simulink model "Vector_xFFT_Ex2"  (R2025a)
settings: Solver=ode45  StartTime=0.0  StopTime=4096/20e3  RelTol=1e-3  EnableMultiTasking=on
undefined symbols (not defined in the file): i, L, vsva1596, xcvc1502
libraries: hdlBasic x7, hdlSSR x5, dspsrcs4 x3, dspxfrm3 x1, vmcUtilities x1
settings Model: Creator=dahlawat  LastModifiedBy=sdegala
settings SolverCC: AlgebraicLoopSolver=TrustRegion
settings DataIOCC: LimitDataPoints=on  SaveFormat=Array  ReturnWorkspaceOutputs=off
settings OptimizationCC: LifeSpan=inf
settings DebuggingCC: UnderspecifiedInitializationDetection=Classic  MergeDetectMultiDrivingBlocksExec=none  SolverPrmCheckMsg=warning  UnconnectedInputMsg=warning  UnconnectedOutputMsg=warning  UnconnectedLineMsg=warning  StateNameClashWarn=warning  SFUnexpectedBacktrackingDiag=warning  SFNoUnconditionalDefaultTransitionDiag=warning  SFExecutionAtInitializationDiag=none  ArithmeticOperatorsInVariantConditions=warning
settings HardwareCC: ProdBitPerPointer=32.0  ProdBitPerSizeT=32.0  ProdBitPerPtrDiffT=32.0  ProdLargestAtomicFloat=None  ProdIntDivRoundTo=Undefined  ProdEndianess=Unspecified  ProdWordSize=32.0  ProdHWDeviceType=32-bit Generic
settings ModelReferenceCC: EnableRefExpFcnMdlSchedulingChecks=on  PropagateSignalLabelsOutOfModel=off
settings SFSimCC: SimUseLocalCustomCode=off  CustomCodeUndefinedFunction=UseInterfaceOnly
settings RTWCC: RTWUseLocalCustomCode=off  GPUComputeCapability=3.5  DLArmComputeVersion=19.05
settings CodeAppCC: StateflowObjectComments=on
settings GRTTargetCC: TargetLangStandard=C89/C90 (ANSI)
settings ConfigComp: CovMetricSettings=dw  CovSaveCumulativeToWorkspaceVar=on  CovSaveSingleToWorkspaceVar=on  CovExternalEMLEnable=off

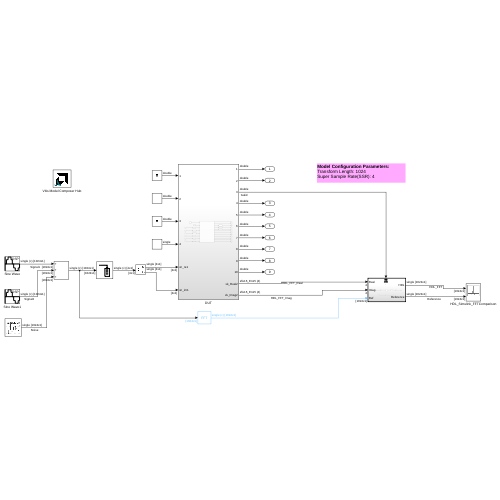
[thumbnail: Simulink's stored preview of the top-level diagram]
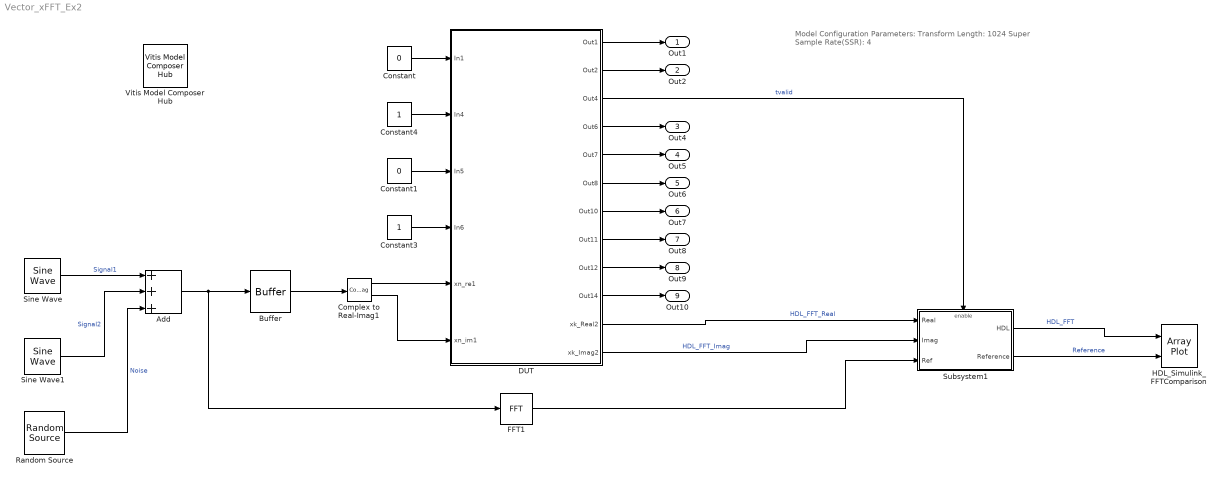
== system Vector_xFFT_Ex2 ==
  note: Model Configuration Parameters:
      | Transform Length: 1024
      | Super Sample Rate(SSR): 4
  Add : Sum  Inputs=+++
  Buffer : Buffer  N=4  OutputFrames=off
  Complex to Real-Imag1 : ComplexToRealImag
  Constant : Constant  Value=0  SampleTime=-1
  Constant1 : Constant  Value=0  SampleTime=-1
  Constant3 : Constant  OutDataTypeStr=single  SampleTime=-1
  Constant4 : Constant  SampleTime=-1
  DUT : Subsystem
  FFT1 : dspxfrm3/FFT  FFTImplementation=FFTW  CompMethod=Table lookup  TableOpt=NEW  TableOptActive=Speed  BitRevOrder=on  Normalize=on  InheritFFTLength=on  FFTLength=64  WrapInput=on  roundingMode=Floor  overflowMode=off  firstCoeffDataTypeStr=Inherit: Same word length as input  firstCoeffLastDataTypeStr=Inherit: Same word length as input  outputMin=[]  outputMax=[]
  HDL_Simulink_FFTComparison : ArrayPlot  NumInputPorts=2  WindowPosition=[1.000000,1.000000,1920.000000,1127.000000,]  Visible=on  ScopeFrameLocation=window  YLimits=[-0.0625 0.5626]  ShowLegend=on
  Random Source : dspsrcs4/Random Source  SrcType=Gaussian  MinVal=0  MaxVal=1  MeanVal=0  VarVal=1e-4  RepMode=Not repeatable  rawSeed=1  IsInherit=off  SampTime=1/20e3  SampFrame=1024  OutComplex=Real  DataType=single  SimulateUsing=Interpreted execution
  Sine Wave : dspsrcs4/Sine Wave  Amplitude=0.5  Frequency=5e3  Phase=0  SampleMode=Discrete  OutComplex=Complex  CompMethod=Trigonometric fcn  TableSize=Speed  SampleTime=1/20e3  SamplesPerFrame=1024  ResetState=Restart at time zero  OutputFrames=off  dataType=single  wordLen=16  udDataType=sfix(16)  fracBitsMode=Best precision  numFracBits=15  OutDataTypeStr=single  LastOutDataTypeStr=single
  Sine Wave1 : dspsrcs4/Sine Wave  Amplitude=0.25  Frequency=15e3  Phase=0  SampleMode=Discrete  OutComplex=Complex  CompMethod=Trigonometric fcn  TableSize=Speed  SampleTime=1/20e3  SamplesPerFrame=1024  ResetState=Restart at time zero  OutputFrames=off  dataType=single  wordLen=16  udDataType=sfix(16)  fracBitsMode=Best precision  numFracBits=15  OutDataTypeStr=single  LastOutDataTypeStr=single
  Subsystem1 : Subsystem
  Vitis Model Composer Hub : vmcUtilities/Vitis Model Composer Hub  Tag=genX  CodeGeneration=off  SubsystemName=DUT  CompilationType=HDLCompilation  ExportTypeV2=IP Catalog  StartColumn=1  NumberOfColumns=1  TargetDirectory=./netlist  exportDesign=off  analyzeDesign=off  validateDesignOnHw=off  ExportType=AI Engines  IpVendor=xilinx.com  IpLibrary=hls  IpVersion=1.0  IpHWLanguage=Verilog  AieCompilerOptions={}  AieSimulatorOptions={}  AieGraphIterations=-1  CreateTestbench=off  TestbenchStackSize=10  RunRtlSim=off  RunCSim=off  RunAieSim=off  AieSimTimeout=50000  RunAieSimProfiling=off  LaunchVitisAnalyzer=off  PlotOutput=off  RunX86Sim=off  X86SimTimeout=10  GenHwImage=off  GenLibadfXo=on  GenHwValidationCode=off  PlatformType=Not Specified  HwSystemType=Baremetal  HwValidationTarget=hw  ProjDevice=xcvc1502-vsva1596-1LHP-i-L  ProjDevicePart=xcvc1502-vsva1596-1LHP-i-L  AIEType=AIE  SamplePeriod=-1  ClockFrequency=200  DataPathParallelism=1  xilinxfamily=versalaicore  part=xcvc1502  speed=-1LHP-i-L  package=vsva1596  directory=./netlist/ip/DUT/src  testbench=off  incr_netlist=off  synthesis_tool=Vivado  clock_wrapper=Clock Enables  dbl_ovrd=According to Block Masks  dcm_input_clock_period=10  sysclk_period=5e4  simulink_period=5e-5  eval_field=0  LogFileName=''  NThreads=4
  Out1 : Outport
  Out2 : Outport  Port=2
  Out4 : Outport  Port=3
  Out5 : Outport  Port=4
  Out6 : Outport  Port=5
  Out7 : Outport  Port=6
  Out8 : Outport  Port=7
  Out9 : Outport  Port=8
  Out10 : Outport  Port=9
  wires:
  Complex to Real-Imag1/2 -> DUT/6(xn_im1)
  DUT/7(Out10) -> Out7/1
  DUT/9(Out12) -> Out9/1
  Constant/1 -> DUT/1(In1)
  Constant1/1 -> DUT/3(In5)
  Subsystem1/1(HDL) -> HDL_Simulink_FFTComparison/1  "HDL_FFT"
  DUT/1(Out1) -> Out1/1
  Constant3/1 -> DUT/4(In6)
  DUT/2(Out2) -> Out2/1
  DUT/10(Out14) -> Out10/1
  DUT/5(Out7) -> Out5/1
  Constant4/1 -> DUT/2(In4)
  DUT/4(Out6) -> Out4/1
  Complex to Real-Imag1/1 -> DUT/5(xn_re1)
  DUT/8(Out11) -> Out8/1
  DUT/6(Out8) -> Out6/1
  DUT/12(xk_Imag2) -> Subsystem1/2(Imag)  "HDL_FFT_Imag"
  DUT/11(xk_Real2) -> Subsystem1/1(Real)  "HDL_FFT_Real"
  DUT/3(Out4) -> Subsystem1/Enable  "tvalid"
  Buffer/1 -> Complex to Real-Imag1/1
  Sine Wave/1 -> Add/1  "Signal1"
  Sine Wave1/1 -> Add/2  "Signal2"
  Add/1 -> FFT1/1, Buffer/1
  Random Source/1 -> Add/3  "Noise"
  FFT1/1 -> Subsystem1/3(Ref)
  Subsystem1/2(Reference) -> HDL_Simulink_FFTComparison/2  "Reference"

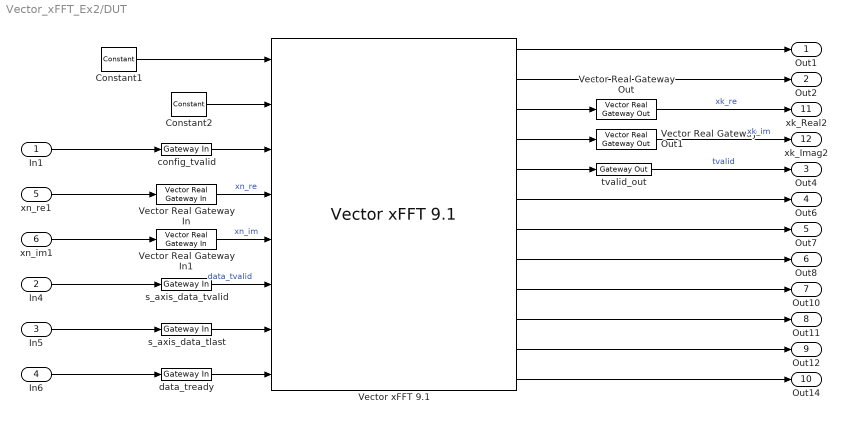
== system Vector_xFFT_Ex2/DUT ==
  In1 : Inport
  In4 : Inport  Port=2
  In5 : Inport  Port=3
  In6 : Inport  Port=4
  xn_re1 : Inport  Port=5
  xn_im1 : Inport  Port=6
  Constant1 : hdlBasic/Constant  const=683  gui_display_data_type=Fixed-point  arith_type=Unsigned  n_bits=10  bin_pt=0  preci_type=Single  exp_width=8  frac_width=24  explicit_period=on  period=1/20e3  XmcBlockStatus=1  maskContainerNames=tabcontainer1  block_type=constant  block_config=sysgen:Constant_config
  Constant2 : hdlBasic/Constant  const=1  gui_display_data_type=Fixed-point  arith_type=Unsigned  n_bits=1  bin_pt=0  preci_type=Single  exp_width=8  frac_width=24  explicit_period=on  period=1/20e3  XmcBlockStatus=1  maskContainerNames=tabcontainer1  block_type=constant  block_config=sysgen:Constant_config
  Vector Real Gateway In : hdlSSR/Vector Real Gateway In  gui_display_data_type=Fixed-point  arith_type=Signed (2's comp)  n_bits=16  bin_pt=15  preci_type=Single  exp_width=8  frac_width=24  quantization="Round  (unbiased: +/- Inf)"  overflow=Saturate  period=1/20e3  sg_ssr=4  UseAsADC=off  ADCChannel='1'  interface=None  automatic_assignment=on  address_offset=hex2dec('00')  intf_name=''  intf_description=''  default_value=0  timing_constraint=None  locs_specified=off  LOCs={}  io_standard={}  inherit_from_input=off  hdl_port=on  interface_prev=1  block_type=realgatewayin_ssr  XmcBlockStatus=1  sg_ssr_prev=4  maskContainerNames=group4  block_width_w=590  block_height_w=670  block_width=640  block_height=850
  Vector Real Gateway In1 : hdlSSR/Vector Real Gateway In  gui_display_data_type=Fixed-point  arith_type=Signed (2's comp)  n_bits=16  bin_pt=15  preci_type=Single  exp_width=8  frac_width=24  quantization="Round  (unbiased: +/- Inf)"  overflow=Saturate  period=1/20e3  sg_ssr=4  UseAsADC=off  ADCChannel='1'  interface=None  automatic_assignment=on  address_offset=hex2dec('00')  intf_name=''  intf_description=''  default_value=0  timing_constraint=None  locs_specified=off  LOCs={}  io_standard={}  inherit_from_input=off  hdl_port=on  interface_prev=1  block_type=realgatewayin_ssr  XmcBlockStatus=1  sg_ssr_prev=4  maskContainerNames=group4  block_width_w=590  block_height_w=670  block_width=640  block_height=850
  Vector Real Gateway Out : hdlSSR/Vector Real Gateway Out  inherit_from_input=on  hdl_port=on  sg_ssr=4  rows=1  columns=1  UseAsDAC=off  DACChannel='1'  interface=None  automatic_assignment=on  address_offset=hex2dec('00')  intf_name=''  intf_description=''  timing_constraint=None  locs_specified=off  LOCs={}  io_standard={}  block_type=realgatewayout_ssr  XmcBlockStatus=1  sg_ssr_prev=4  maskContainerNames=group4  block_width_w=590  block_height_w=620  block_width=620  block_height=750
  Vector Real Gateway Out1 : hdlSSR/Vector Real Gateway Out  inherit_from_input=on  hdl_port=on  sg_ssr=4  rows=1  columns=1  UseAsDAC=off  DACChannel='1'  interface=None  automatic_assignment=on  address_offset=hex2dec('00')  intf_name=''  intf_description=''  timing_constraint=None  locs_specified=off  LOCs={}  io_standard={}  block_type=realgatewayout_ssr  XmcBlockStatus=1  sg_ssr_prev=4  maskContainerNames=group4  block_width_w=590  block_height_w=620  block_width=620  block_height=750
  Vector xFFT 9.1 : hdlSSR/Vector xFFT 9.1  transform_length=1024  target_clock_frequency=250  target_data_throughput=50  implementation_options=automatically_select  run_time_configurable_transform_length=off  enable_ssr=off  super_sample_rates=4  phase_factor_width=24  scaling_options=scaled  rounding_modes=truncation  aclken=off  aresetn=off  output_ordering=bit_reversed_order  cyclic_prefix_insertion=off  throttle_scheme=nonrealtime  xk_index=off  ovflo=off  trim_axipin_name=on  memory_options_data=block_ram  memory_options_phase_factors=block_ram  number_of_stages_using_block_ram_for_data_and_phase_factors=2  memory_options_reorder=block_ram  memory_options_hybrid=off  complex_mult_type=use_mults_resources  butterfly_type=use_luts  simulation_type=hybrid_sim  ip_name=Fast Fourier Transform  ip_version=9.1  block_type=fast_fourier_transform_v9_1_ssr  XmcBlockStatus=1  ssr_prev=4  scaling_options_prev=scaled  throttle_scheme_prev=nonrealtime  ovflo_prev=off
      settings: block_version=1.0
  config_tvalid : hdlBasic/Gateway In  gui_display_data_type=Boolean  arith_type=Boolean  n_bits=16  bin_pt=15  preci_type=Single  exp_width=8  frac_width=24  rows=1  columns=1  quantization="Round  (unbiased: +/- Inf)"  overflow=Saturate  period=1/20e3  UseAsADC=off  ADCChannel='1'  interface=None  automatic_assignment=on  address_offset=hex2dec('00')  intf_name=''  intf_description=''  default_value=0  timing_constraint=None  locs_specified=off  LOCs={}  io_standard={}  inherit_from_input=off  hdl_port=on  XmcBlockStatus=1  maskContainerNames=group4  block_type=gatewayin  block_config=sysgen:gateway_in_config  block_width_w=590  block_height_w=620  block_width=640  block_height=850
  data_tready : hdlBasic/Gateway In  gui_display_data_type=Boolean  arith_type=Boolean  n_bits=16  bin_pt=15  preci_type=Single  exp_width=8  frac_width=24  rows=1  columns=1  quantization="Round  (unbiased: +/- Inf)"  overflow=Saturate  period=1/20e3  UseAsADC=off  ADCChannel='1'  interface=None  automatic_assignment=on  address_offset=hex2dec('00')  intf_name=''  intf_description=''  default_value=0  timing_constraint=None  locs_specified=off  LOCs={}  io_standard={}  inherit_from_input=off  hdl_port=on  XmcBlockStatus=1  maskContainerNames=group4  block_type=gatewayin  block_config=sysgen:gateway_in_config  block_width_w=590  block_height_w=620  block_width=640  block_height=850
  s_axis_data_tlast : hdlBasic/Gateway In  gui_display_data_type=Boolean  arith_type=Boolean  n_bits=9  bin_pt=8  preci_type=Single  exp_width=8  frac_width=24  rows=1  columns=1  quantization="Round  (unbiased: +/- Inf)"  overflow=Saturate  period=1/20e3  UseAsADC=off  ADCChannel='1'  interface=None  automatic_assignment=on  address_offset=hex2dec('00')  intf_name=''  intf_description=''  default_value=0  timing_constraint=None  locs_specified=off  LOCs={}  io_standard={}  inherit_from_input=off  hdl_port=on  XmcBlockStatus=1  maskContainerNames=group4  block_type=gatewayin  block_config=sysgen:gateway_in_config  block_width_w=590  block_height_w=620  block_width=640  block_height=850
  s_axis_data_tvalid : hdlBasic/Gateway In  gui_display_data_type=Boolean  arith_type=Boolean  n_bits=9  bin_pt=8  preci_type=Single  exp_width=8  frac_width=24  rows=1  columns=1  quantization="Round  (unbiased: +/- Inf)"  overflow=Saturate  period=1/20e3  UseAsADC=off  ADCChannel='1'  interface=None  automatic_assignment=on  address_offset=hex2dec('00')  intf_name=''  intf_description=''  default_value=0  timing_constraint=None  locs_specified=off  LOCs={}  io_standard={}  inherit_from_input=off  hdl_port=on  XmcBlockStatus=1  maskContainerNames=group4  block_type=gatewayin  block_config=sysgen:gateway_in_config  block_width_w=590  block_height_w=620  block_width=640  block_height=850
  tvalid_out : hdlBasic/Gateway Out  inherit_from_input=off  bool_to_boolean=off  hdl_port=on  rows=1  columns=1  UseAsDAC=off  DACChannel='1'  interface=None  automatic_assignment=on  address_offset=hex2dec('00')  intf_name=''  intf_description=''  timing_constraint=None  locs_specified=off  LOCs={}  io_standard={}  XmcBlockStatus=1  maskContainerNames=group4  block_type=gatewayout  block_config=sysgen:gateway_out_config  block_width_w=590  block_height_w=620  block_width=620  block_height=750
  Out1 : Outport
  Out2 : Outport  Port=2
  Out4 : Outport  Port=3
  Out6 : Outport  Port=4
  Out7 : Outport  Port=5
  Out8 : Outport  Port=6
  Out10 : Outport  Port=7
  Out11 : Outport  Port=8
  Out12 : Outport  Port=9
  Out14 : Outport  Port=10
  xk_Real2 : Outport  Port=11
  xk_Imag2 : Outport  Port=12
  wires:
  config_tvalid/1 -> Vector xFFT 9.1/3
  Vector Real Gateway Out/1 -> xk_Real2/1  "xk_re"
  In6/1 -> data_tready/1
  Vector Real Gateway Out1/1 -> xk_Imag2/1  "xk_im"
  In4/1 -> s_axis_data_tvalid/1
  In1/1 -> config_tvalid/1
  Vector xFFT 9.1/2 -> Out2/1
  Constant2/1 -> Vector xFFT 9.1/2
  Vector xFFT 9.1/1 -> Out1/1
  Vector xFFT 9.1/11 -> Out12/1
  In5/1 -> s_axis_data_tlast/1
  xn_re1/1 -> Vector Real Gateway In/1
  xn_im1/1 -> Vector Real Gateway In1/1
  s_axis_data_tvalid/1 -> Vector xFFT 9.1/6  "data_tvalid"
  Vector xFFT 9.1/6 -> Out6/1
  Vector xFFT 9.1/7 -> Out7/1
  Vector xFFT 9.1/8 -> Out8/1
  Vector xFFT 9.1/9 -> Out10/1
  Vector xFFT 9.1/10 -> Out11/1
  Vector Real Gateway In1/1 -> Vector xFFT 9.1/5  "xn_im"
  Vector Real Gateway In/1 -> Vector xFFT 9.1/4  "xn_re"
  Vector xFFT 9.1/3 -> Vector Real Gateway Out/1
  s_axis_data_tlast/1 -> Vector xFFT 9.1/7
  data_tready/1 -> Vector xFFT 9.1/8
  Vector xFFT 9.1/5 -> tvalid_out/1
  tvalid_out/1 -> Out4/1  "tvalid"
  Vector xFFT 9.1/4 -> Vector Real Gateway Out1/1
  Vector xFFT 9.1/12 -> Out14/1
  Constant1/1 -> Vector xFFT 9.1/1

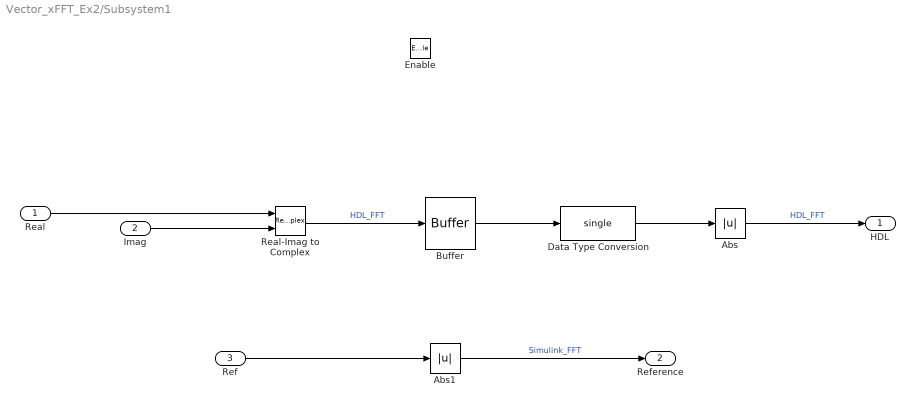
== system Vector_xFFT_Ex2/Subsystem1 ==
  Real : Inport
  Imag : Inport  Port=2
  Ref : Inport  Port=3
  Enable : EnablePort
  Abs : Abs  SaturateOnIntegerOverflow=off
  Abs1 : Abs  SaturateOnIntegerOverflow=off
  Buffer : Buffer  N=1024  OutputFrames=off
  Data Type Conversion : DataTypeConversion  OutDataTypeStr=single  SaturateOnIntegerOverflow=off  RndMeth=Floor
  Real-Imag to Complex : RealImagToComplex
  HDL : Outport
  Reference : Outport  Port=2
  wires:
  Real-Imag to Complex/1 -> Buffer/1  "HDL_FFT"
  Imag/1 -> Real-Imag to Complex/2
  Real/1 -> Real-Imag to Complex/1
  Abs/1 -> HDL/1  "HDL_FFT"
  Buffer/1 -> Data Type Conversion/1
  Data Type Conversion/1 -> Abs/1
  Ref/1 -> Abs1/1
  Abs1/1 -> Reference/1  "Simulink_FFT"
